simulink model "Lab_Bai1_GioiThieu_2019a"  (R2019a)
settings: Solver=VariableStepAuto  StartTime=0.0  StopTime=10.0  RelTol=1e-3
undefined symbols (not defined in the file): randsrc
libraries: commrandsrc3 x2, dsparch4 x1
settings Model: Creator=Thanh_Hai  LastModifiedBy=Thanh_Hai

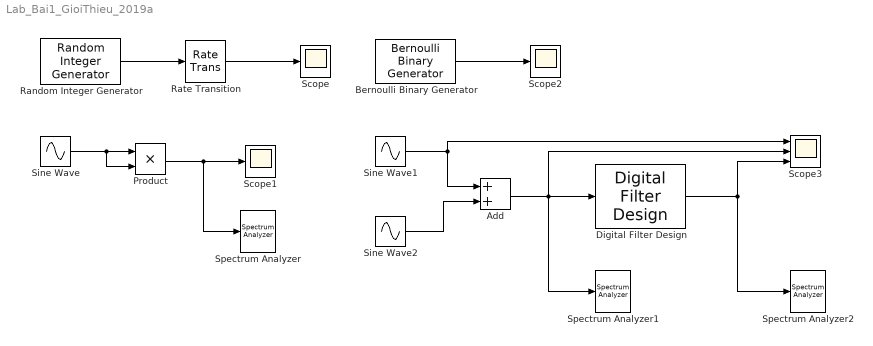
== system Lab_Bai1_GioiThieu_2019a ==
  Add : Sum
  Bernoulli Binary Generator : commrandsrc3/Bernoulli Binary Generator  ProbabilityOfZero=0.5  SeedSource=Parameter  Seed=randsrc(1,1,[1:100])  SampleTime=1  SamplesPerFrame=1  OutputDataType=double  SimulateUsing=Interpreted execution
      settings: SourceProductName=Communications Toolbox
  Digital Filter Design : dsparch4/Digital Filter Design  mwdsp_browser_bugfix_var=off
  Product : Product
  Random Integer Generator : commrandsrc3/Random Integer Generator  SetSize=8  SeedSource=Auto  Seed=0  SampleTime=1  SamplesPerFrame=2  OutputDataType=double  SimulateUsing=Interpreted execution
      settings: SourceProductName=Communications Toolbox
  Rate Transition : RateTransition
  Scope : Scope
  Scope1 : Scope
  Scope2 : Scope
  Scope3 : Scope  NumInputPorts=3
  Sine Wave : Sin  Frequency=2*pi*1000  SampleTime=1/10000
  Sine Wave1 : Sin  Frequency=2*pi*1000  SampleTime=1/50000
  Sine Wave2 : Sin  Frequency=2*pi*3000  SampleTime=1/50000
  Spectrum Analyzer : SpectrumAnalyzer
  Spectrum Analyzer1 : SpectrumAnalyzer
  Spectrum Analyzer2 : SpectrumAnalyzer
  wires:
  Random Integer Generator/1 -> Rate Transition/1
  Rate Transition/1 -> Scope/1
  Bernoulli Binary Generator/1 -> Scope2/1
  Sine Wave/1 -> Product/2, Product/1
  Product/1 -> Spectrum Analyzer/1, Scope1/1
  Sine Wave1/1 -> Scope3/1, Add/1
  Sine Wave2/1 -> Add/2
  Add/1 -> Spectrum Analyzer1/1, Scope3/2, Digital Filter Design/1
  Digital Filter Design/1 -> Spectrum Analyzer2/1, Scope3/3
